simulink model "Quadrotor_Sensor_Convert"  (Simulink 7.6)
settings: Solver=FixedStepDiscrete  StartTime=0.0  StopTime=10.0  FixedStep=0.1  RelTol=1e-3
settings Model: Creator=jporter  LastModifiedBy=Administrator
settings DataIOCC: LimitDataPoints=off  SaveOutput=off  SignalLogging=off  DSMLogging=off  SaveTime=off
settings OptimizationCC: InlineParams=on  EnhancedBackFolding=on  PassReuseOutputArgsAs=Individual arguments  OptimizeModelRefInitCode=on
settings HardwareCC: ProdLargestAtomicInteger=Long  ProdLargestAtomicFloat=Float  ProdIntDivRoundTo=Floor  ProdEndianess=LittleEndian  ProdHWDeviceType=ARM Compatible->ARM 7  TargetLargestAtomicInteger=Long  TargetLargestAtomicFloat=Float  TargetIntDivRoundTo=Floor  TargetEndianess=LittleEndian  TargetHWDeviceType=ARM Compatible->ARM 7
settings RTWCC: SystemTargetFile=ert.tlc  GenCodeOnly=on  TemplateMakefile=ert_default_tmf  Description=Real-Time Workshop Embedded Coder  GenerateReport=on  ProcessScript=ert_make_rtw_hook  IncludeHyperlinkInReport=on  LaunchReport=on  GenerateTraceReportSl=on  GenerateTraceReportEml=on  RTWCompilerOptimization=On  CheckMdlBeforeBuild=Warning
settings CodeAppCC: IgnoreCustomStorageClasses=off
settings ERTTargetCC: MultiwordLength=2048  GenerateSampleERTMain=on  CombineSignalStateStructs=on  MultiInstanceERTCode=on  SupportNonFinite=off  SupportComplex=off  MultiInstanceErrorCode=Warning  ERTCustomFileTemplate=example_file_process.tlc

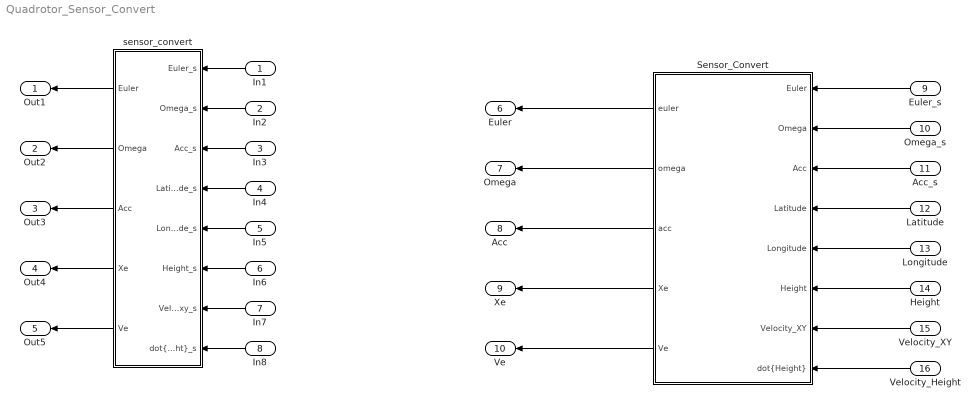
== system Quadrotor_Sensor_Convert ==
  In1 : Inport  OutDataTypeStr=single  PortDimensions=[3]
  In2 : Inport  Port=2  OutDataTypeStr=single  PortDimensions=[3]
  In3 : Inport  Port=3  OutDataTypeStr=single  PortDimensions=[3]
  In4 : Inport  Port=4  OutDataTypeStr=single  PortDimensions=[1]
  In5 : Inport  Port=5  OutDataTypeStr=single  PortDimensions=[1]
  In6 : Inport  Port=6  OutDataTypeStr=single  PortDimensions=[1]
  In7 : Inport  Port=7  OutDataTypeStr=single  PortDimensions=[2]
  In8 : Inport  Port=8  OutDataTypeStr=single  PortDimensions=[1]
  Euler_s : Inport  Port=9  OutDataTypeStr=single  PortDimensions=[3]
  Omega_s : Inport  Port=10  OutDataTypeStr=single  PortDimensions=[3]
  Acc_s : Inport  Port=11  OutDataTypeStr=single  PortDimensions=[3]
  Latitude : Inport  Port=12  OutDataTypeStr=single  PortDimensions=[1]
  Longitude : Inport  Port=13  OutDataTypeStr=single  PortDimensions=[1]
  Height : Inport  Port=14  OutDataTypeStr=single  PortDimensions=[1]
  Velocity_XY : Inport  Port=15  OutDataTypeStr=single  PortDimensions=[2]
  Velocity_Height : Inport  Port=16  OutDataTypeStr=single  PortDimensions=[1]
  Sensor_Convert : Subsystem
  sensor_convert : Subsystem
  Out1 : Outport
  Out2 : Outport  Port=2
  Out3 : Outport  Port=3
  Out4 : Outport  Port=4
  Out5 : Outport  Port=5
  Euler : Outport  Port=6
  Omega : Outport  Port=7
  Acc : Outport  Port=8
  Xe : Outport  Port=9
  Ve : Outport  Port=10
  wires:
  In1/1 -> sensor_convert/1(Euler_s)
  In2/1 -> sensor_convert/2(Omega_s)
  In3/1 -> sensor_convert/3(Acc_s)
  In4/1 -> sensor_convert/4(Latitude_s)
  In5/1 -> sensor_convert/5(Longitude_s)
  In6/1 -> sensor_convert/6(Height_s)
  In7/1 -> sensor_convert/7(Velocity_xy_s)
  In8/1 -> sensor_convert/8("dot{Height}_s")
  sensor_convert/1(Euler) -> Out1/1
  sensor_convert/2(Omega) -> Out2/1
  sensor_convert/3(Acc) -> Out3/1
  sensor_convert/4(Xe) -> Out4/1
  sensor_convert/5(Ve) -> Out5/1
  Sensor_Convert/1(euler) -> Euler/1
  Euler_s/1 -> Sensor_Convert/1(Euler)
  Omega_s/1 -> Sensor_Convert/2(Omega)
  Acc_s/1 -> Sensor_Convert/3(Acc)
  Latitude/1 -> Sensor_Convert/4(Latitude)
  Longitude/1 -> Sensor_Convert/5(Longitude)
  Height/1 -> Sensor_Convert/6(Height)
  Velocity_XY/1 -> Sensor_Convert/7(Velocity_XY)
  Velocity_Height/1 -> Sensor_Convert/8("dot{Height}")
  Sensor_Convert/2(omega) -> Omega/1
  Sensor_Convert/3(acc) -> Acc/1
  Sensor_Convert/4(Xe) -> Xe/1
  Sensor_Convert/5(Ve) -> Ve/1

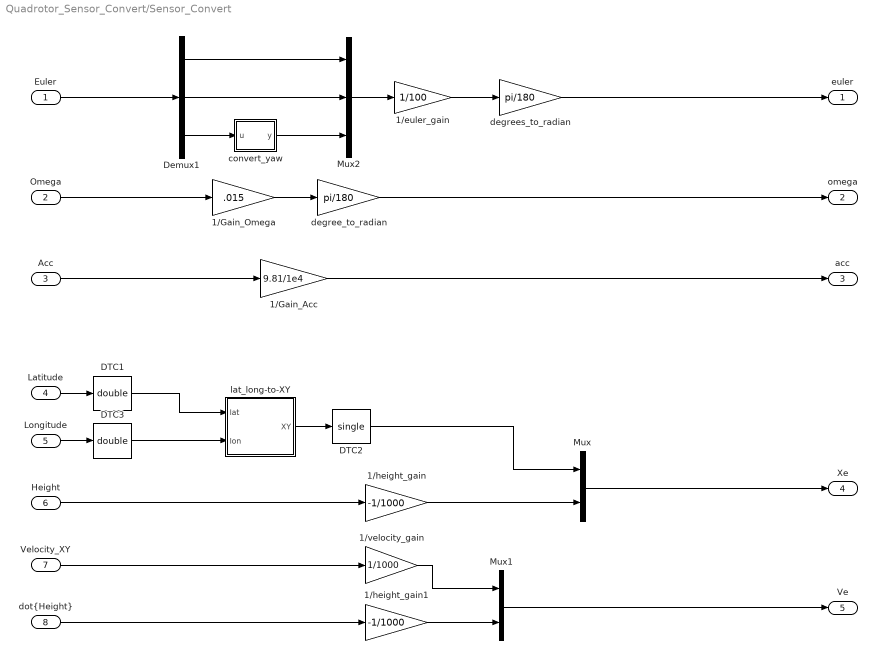
== system Quadrotor_Sensor_Convert/Sensor_Convert ==
  Euler : Inport
  Omega : Inport  Port=2
  Acc : Inport  Port=3
  Latitude : Inport  Port=4  OutDataTypeStr=single
  Longitude : Inport  Port=5  OutDataTypeStr=single
  Height : Inport  Port=6  OutDataTypeStr=single
  Velocity_XY : Inport  Port=7  OutDataTypeStr=single
  "dot{Height}" : Inport  Port=8  OutDataTypeStr=single
  1/Gain_Acc : Gain  Gain=9.81/1e4  OutDataTypeStr=single
  1/Gain_Omega : Gain  Gain=.015  OutDataTypeStr=single
  1/euler_gain : Gain  Gain=1/100
  1/height_gain : Gain  Gain=-1/1000
  1/height_gain1 : Gain  Gain=-1/1000
  1/velocity_gain : Gain  Gain=1/1000
  DTC1 : DataTypeConversion  OutDataTypeStr=double
  DTC2 : DataTypeConversion  OutDataTypeStr=single
  DTC3 : DataTypeConversion  OutDataTypeStr=double
  Demux1 : Demux  Outputs=3
  Mux : Mux  Inputs=[2,1]
  Mux1 : Mux  Inputs=[2,1]
  Mux2 : Mux  Inputs=3
  convert_yaw : Stateflow chart  TreatAsAtomicUnit=on
  degree_to_radian : Gain  Gain=pi/180  OutDataTypeStr=single
  degrees_to_radian : Gain  Gain=pi/180  OutDataTypeStr=single
  lat_long-to-XY : Stateflow chart  TreatAsAtomicUnit=on
  euler : Outport
  omega : Outport  Port=2
  acc : Outport  Port=3
  Xe : Outport  Port=4
  Ve : Outport  Port=5
  wires:
  Velocity_XY/1 -> 1/velocity_gain/1
  Height/1 -> 1/height_gain/1
  1/height_gain/1 -> Mux/2
  Latitude/1 -> DTC1/1
  Longitude/1 -> DTC3/1
  lat_long-to-XY/1(XY) -> DTC2/1
  Mux/1 -> Xe/1
  "dot{Height}"/1 -> 1/height_gain1/1
  1/height_gain1/1 -> Mux1/2
  Mux1/1 -> Ve/1
  DTC2/1 -> Mux/1
  1/velocity_gain/1 -> Mux1/1
  DTC1/1 -> lat_long-to-XY/1(lat)
  DTC3/1 -> lat_long-to-XY/2(lon)
  Omega/1 -> 1/Gain_Omega/1
  1/Gain_Omega/1 -> degree_to_radian/1
  1/Gain_Acc/1 -> acc/1
  Acc/1 -> 1/Gain_Acc/1
  degree_to_radian/1 -> omega/1
  Euler/1 -> Demux1/1
  Mux2/1 -> 1/euler_gain/1
  degrees_to_radian/1 -> euler/1
  1/euler_gain/1 -> degrees_to_radian/1
  Demux1/1 -> Mux2/1
  Demux1/2 -> Mux2/2
  convert_yaw/1(y) -> Mux2/3
  Demux1/3 -> convert_yaw/1(u)

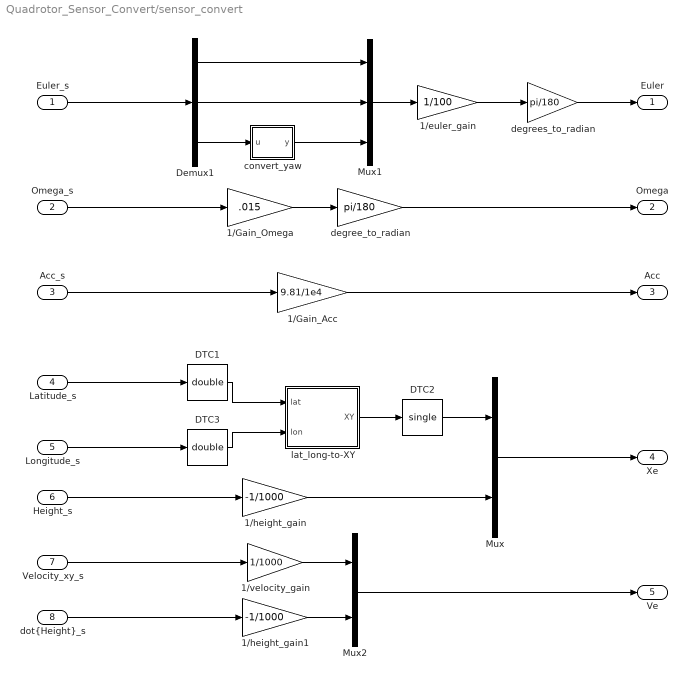
== system Quadrotor_Sensor_Convert/sensor_convert ==
  Euler_s : Inport
  Omega_s : Inport  Port=2
  Acc_s : Inport  Port=3
  Latitude_s : Inport  Port=4
  Longitude_s : Inport  Port=5
  Height_s : Inport  Port=6  OutDataTypeStr=single
  Velocity_xy_s : Inport  Port=7  OutDataTypeStr=single
  "dot{Height}_s" : Inport  Port=8  OutDataTypeStr=single
  1/Gain_Acc : Gain  Gain=9.81/1e4  OutDataTypeStr=single
  1/Gain_Omega : Gain  Gain=.015  OutDataTypeStr=single
  1/euler_gain : Gain  Gain=1/100
  1/height_gain : Gain  Gain=-1/1000
  1/height_gain1 : Gain  Gain=-1/1000
  1/velocity_gain : Gain  Gain=1/1000
  DTC1 : DataTypeConversion  OutDataTypeStr=double
  DTC2 : DataTypeConversion  OutDataTypeStr=single
  DTC3 : DataTypeConversion  OutDataTypeStr=double
  Demux1 : Demux  Outputs=3
  Mux : Mux  Inputs=[2,1]
  Mux1 : Mux  Inputs=3
  Mux2 : Mux  Inputs=[2,1]
  convert_yaw : Stateflow chart  TreatAsAtomicUnit=on
  degree_to_radian : Gain  Gain=pi/180  OutDataTypeStr=single
  degrees_to_radian : Gain  Gain=pi/180  OutDataTypeStr=single
  lat_long-to-XY : Stateflow chart  TreatAsAtomicUnit=on
  Euler : Outport
  Omega : Outport  Port=2
  Acc : Outport  Port=3
  Xe : Outport  Port=4
  Ve : Outport  Port=5
  wires:
  Omega_s/1 -> 1/Gain_Omega/1
  1/Gain_Omega/1 -> degree_to_radian/1
  1/Gain_Acc/1 -> Acc/1
  Acc_s/1 -> 1/Gain_Acc/1
  degree_to_radian/1 -> Omega/1
  Euler_s/1 -> Demux1/1
  Mux1/1 -> 1/euler_gain/1
  degrees_to_radian/1 -> Euler/1
  1/euler_gain/1 -> degrees_to_radian/1
  Demux1/1 -> Mux1/1
  Demux1/2 -> Mux1/2
  convert_yaw/1(y) -> Mux1/3
  Demux1/3 -> convert_yaw/1(u)
  Velocity_xy_s/1 -> 1/velocity_gain/1
  Height_s/1 -> 1/height_gain/1
  1/height_gain/1 -> Mux/2
  Latitude_s/1 -> DTC1/1
  Longitude_s/1 -> DTC3/1
  lat_long-to-XY/1(XY) -> DTC2/1
  Mux/1 -> Xe/1
  "dot{Height}_s"/1 -> 1/height_gain1/1
  1/height_gain1/1 -> Mux2/2
  Mux2/1 -> Ve/1
  DTC2/1 -> Mux/1
  1/velocity_gain/1 -> Mux2/1
  DTC1/1 -> lat_long-to-XY/1(lat)
  DTC3/1 -> lat_long-to-XY/2(lon)

== matlab function Sensor_Convert/lat_long-to-XY ==
  data: XY output double size=[2]; lat input double size=[1]; lon input double size=[1]
function XY  = fcn(lat,lon)
%Convert latitude and longitude to relative XY position from an initial
%latitude and longitude reading
    persistent lat_0;
    persistent lon_0;
    R = 6371e3;         %Earth's Radius meters
    lat = lat*pi/180e7; %Convert from 1e-7 degrees to radians
    lon = lon*pi/180e7; %Convert from 1e-7 degrees to radians
    if isempty(lat_0)
        lat_0 = lat;
    end
    if lat_0 == 0
        lat_0 = lat;
    end
    if isempty(lon_0)
        lon_0 = lon;
    end
    if lon_0 == 0
        lon_0 = lon;
    end
    XY = zeros(2,1);
    if (lat_0 ~= 0) && (lon_0 ~= 0)
        %Compute distance between two-points using haversine formula
        del_lat = lat - lat_0;
        del_lon = lon - lon_0;
        a = sin(del_lat/2)^2 + cos(lat)*sin(del_lon/2)^2;
        c = 2*atan2(sqrt(a),sqrt(1-a));
        d = R*c;     %Distance traveled from starting point (0,0) in meters
        yt = sin(del_lon)*cos(lat);
        xt = cos(lat_0)*sin(lat) - sin(lat_0)*cos(lat)*cos(del_lon);
        th = atan2(yt,xt);
        X = d*cos(th);
        Y = d*sin(th);
        XY(1) = X;
        XY(2) = Y;
    end

== matlab function Sensor_Convert/convert_yaw ==
  data: u input double; y output double
function y = fcn(u)
    euler_gain = 100;
    if u > 180*euler_gain
        y = u - 360*euler_gain;
    else
        y = u;
    end

== matlab function sensor_convert/convert_yaw ==
  data: u input double; y output double
function y = fcn(u)
    euler_gain = 100;
    if u > 180*euler_gain
        y = u - 360*euler_gain;
    else
        y = u;
    end

== matlab function sensor_convert/lat_long-to-XY ==
  data: XY output double size=[2]; lat input double size=[1]; lon input double size=[1]
function XY  = fcn(lat,lon)
%Convert latitude and longitude to relative XY position from an initial
%latitude and longitude reading
    persistent lat_0;
    persistent lon_0;
    R = 6371e3;         %Earth's Radius meters
    lat = lat*pi/180e7; %Convert from 1e-7 degrees to radians
    lon = lon*pi/180e7; %Convert from 1e-7 degrees to radians
    if isempty(lat_0)
        lat_0 = lat;
    end
    if lat_0 == 0
        lat_0 = lat;
    end
    if isempty(lon_0)
        lon_0 = lon;
    end
    if lon_0 == 0
        lon_0 = lon;
    end
    XY = zeros(2,1);
    if (lat_0 ~= 0) && (lon_0 ~= 0)
        %Compute distance between two-points using haversine formula
        del_lat = lat - lat_0;
        del_lon = lon - lon_0;
        a = sin(del_lat/2)^2 + cos(lat)*sin(del_lon/2)^2;
        c = 2*atan2(sqrt(a),sqrt(1-a));
        d = R*c;     %Distance traveled from starting point (0,0) in meters
        yt = sin(del_lon)*cos(lat);
        xt = cos(lat_0)*sin(lat) - sin(lat_0)*cos(lat)*cos(del_lon);
        th = atan2(yt,xt);
        X = d*cos(th);
        Y = d*sin(th);
        XY(1) = X;
        XY(2) = Y;
    end
    
    lat0 = lat_0;
    lon0 = lon_0;
